simulink model "Proposed DTC"  (R2022a)
settings: Solver=ode1  StartTime=0.0  StopTime=Inf  FixedStep=Ts  RelTol=1e-3  EnableMultiTasking=on
PostLoadFcn:
  | , if any(exist('dsrtsu_mdlpostloadfcn', 'file') ~= 0), dsrtsu_mdlpostloadfcn('Execute', bdroot); end,
InitFcn:
  | , if any(exist('rtifpga_mdlclblib', 'file') ~= 0), rtifpga_mdlclblib('Init', bdroot); end,
undefined symbols (not defined in the file): P, Ts
libraries: rtilib1104 x15, rtitasklib x1
(part 1 of 2)
settings Model: DSRTSU_INTERNAL_RTI_VER=600  DSRTSU_INTERNAL_RTI_TYPE=rti1104  DSRTSU_INTERNAL_RTIFPGA=180  DSRTSU_INTERNAL_RTISTBM_VER=1.4.4  Creator=Admin  LastModifiedBy=acer
settings SolverCC: AlgebraicLoopSolver=TrustRegion
settings DataIOCC: LimitDataPoints=on  SaveFormat=Array  SignalLoggingSaveFormat=ModelDataLogs  ReturnWorkspaceOutputs=off
settings OptimizationCC: BlockReduction=off  ConditionallyExecuteInputs=off  OptimizeBlockIOStorage=off  BufferReuse=off  GlobalBufferReuse=off  ExpressionFolding=off  ExpressionDepthLimit=2147483647  LocalBlockOutputs=off  LifeSpan=inf
settings DebuggingCC: UnderspecifiedInitializationDetection=Classic  MergeDetectMultiDrivingBlocksExec=none  SolverPrmCheckMsg=warning  MultiTaskDSMMsg=warning  MultiTaskCondExecSysMsg=none  FcnCallInpInsideContextMsg=warning  UnconnectedInputMsg=warning  UnconnectedOutputMsg=warning  UnconnectedLineMsg=warning  StateNameClashWarn=warning  SFUnexpectedBacktrackingDiag=warning  SFNoUnconditionalDefaultTransitionDiag=warning  SFExecutionAtInitializationDiag=none  SFMachineParentedDataDiag=warning  ArithmeticOperatorsInVariantConditions=warning
settings HardwareCC: ProdBitPerPointer=32  ProdBitPerSizeT=32  ProdBitPerPtrDiffT=32  ProdLargestAtomicInteger=Integer  ProdEndianess=BigEndian  ProdWordSize=32  ProdHWDeviceType=Custom Processor->Custom  TargetIntDivRoundTo=Zero  TargetEndianess=BigEndian  TargetHWDeviceType=Custom Processor->Custom
settings ModelReferenceCC: PropagateSignalLabelsOutOfModel=off
settings SFSimCC: SimUseLocalCustomCode=off  MATLABDynamicMemAlloc=off  CustomCodeUndefinedFunction=UseInterfaceOnly
settings RTWCC: Description=dSPACE DS1104 Hardware Platform  SystemTargetFile=rti1104.tlc  MakeCommand=make_rti  TemplateMakefile=rti1104.tmf  RTWUseLocalCustomCode=off
settings CodeAppCC: StateflowObjectComments=on
settings STFCustomTargetCC: ParMdlRefBuildCompliant=on  GRTInterface=off  SystemTargetFile=rti1104.tlc
settings GRTTargetCC: TargetLangStandard=C89/C90 (ANSI)  CompOptLevelCompliant=off  ConcurrentExecutionCompliant=off  CombineOutputUpdateFcns=off  MatFileLogging=off  CPPClassGenCompliant=off  UseToolchainInfoCompliant=off  ExtModeMexFile=noextcomm
settings ConfigComp: CovMetricSettings=dw  CovSaveCumulativeToWorkspaceVar=on  CovSaveSingleToWorkspaceVar=on  CovExternalEMLEnable=off

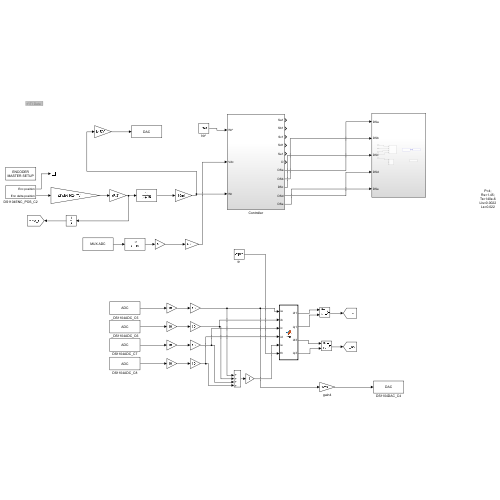
[thumbnail: Simulink's stored preview of the top-level diagram]
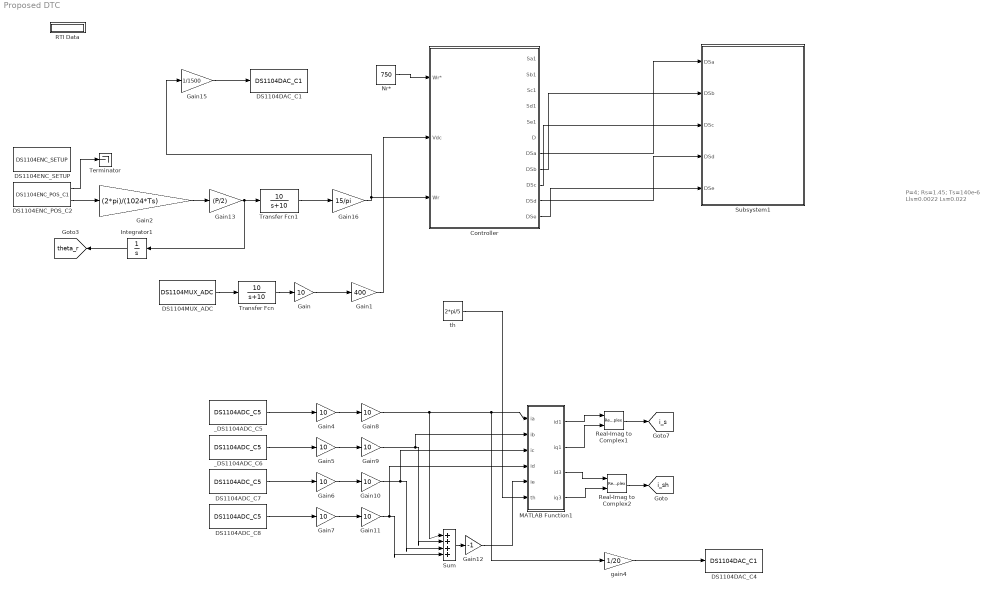
== system Proposed DTC ==
  note: P=4;
      | Rs=1.45;
      | Ts=140e-6
      | Lls=0.0022
      | Ls=0.022
  Controller : Subsystem
  DS1104ADC_C7 : rtilib1104/DS1104 MASTER PPC/DS1104ADC_C5  ChannelNo=7  TriggerMode=0  Reserved1=[]  Reserved2=[]  Reserved3=[]  Reserved4=[]  DialogFcn=gui1104adc  UnitName={ 'DS1104ADC_C' }  UnitValues={ 7 }  DSProperties=struct('RTI',struct('Version',uint32(1),'BlockType',struct('isSLSource',uint8(1),'isSLSink',uint8(0),'isHWSource',uint8(1),'isHWSink',uint8(0),'isSetup',uint8(0),'isInline',uint8(1),'isNonInline',uint8(0),'isInterrupt',uint8(0),'isChannelwise',uint8(1)),'IOBoardType','DS1104MASTER','UnitType','ADC','Identifier','ADC','DialogType','ML','BlockSet','NONE','SlaveProcessor','NONE'))
      settings: SourceProductName=dSPACE RTI1104
  DS1104ADC_C8 : rtilib1104/DS1104 MASTER PPC/DS1104ADC_C5  ChannelNo=8  TriggerMode=0  Reserved1=[]  Reserved2=[]  Reserved3=[]  Reserved4=[]  DialogFcn=gui1104adc  UnitName={ 'DS1104ADC_C' }  UnitValues={ 8 }  DSProperties=struct('RTI',struct('Version',uint32(1),'BlockType',struct('isSLSource',uint8(1),'isSLSink',uint8(0),'isHWSource',uint8(1),'isHWSink',uint8(0),'isSetup',uint8(0),'isInline',uint8(1),'isNonInline',uint8(0),'isInterrupt',uint8(0),'isChannelwise',uint8(1)),'IOBoardType','DS1104MASTER','UnitType','ADC','Identifier','ADC','DialogType','ML','BlockSet','NONE','SlaveProcessor','NONE'))
      settings: SourceProductName=dSPACE RTI1104
  DS1104DAC_C1 : rtilib1104/DS1104 MASTER PPC/DS1104DAC_C1  ChannelNo=1  InitValue=0  TermMode=0  TermValue=0  Reserved1=[]  Reserved2=[]  Reserved3=[]  Reserved4=[]  DialogFcn=gui1104dac  UnitName={ 'DS1104DAC_C'}  UnitValues={ 1 }  DSProperties=struct('RTI',struct('Version',uint32(1),'BlockType',struct('isSLSource',uint8(0),'isSLSink',uint8(1),'isHWSource',uint8(0),'isHWSink',uint8(1),'isSetup',uint8(0),'isInline',uint8(1),'isNonInline',uint8(0),'isInterrupt',uint8(0),'isChannelwise',uint8(1)),'IOBoardType','DS1104MASTER','UnitType','DAC','Identifier','DAC','DialogType','ML','BlockSet','NONE','SlaveProcessor','NONE'))
      settings: SourceProductName=dSPACE RTI1104
  DS1104DAC_C4 : rtilib1104/DS1104 MASTER PPC/DS1104DAC_C1  ChannelNo=4  InitValue=0  TermMode=0  TermValue=0  Reserved1=[]  Reserved2=[]  Reserved3=[]  Reserved4=[]  DialogFcn=gui1104dac  UnitName={ 'DS1104DAC_C'}  UnitValues={4}  DSProperties=struct('RTI',struct('Version',uint32(1),'BlockType',struct('isSLSource',uint8(0),'isSLSink',uint8(1),'isHWSource',uint8(0),'isHWSink',uint8(1),'isSetup',uint8(0),'isInline',uint8(1),'isNonInline',uint8(0),'isInterrupt',uint8(0),'isChannelwise',uint8(1)),'IOBoardType','DS1104MASTER','UnitType','DAC','Identifier','DAC','DialogType','ML','BlockSet','NONE','SlaveProcessor','NONE'))
      settings: SourceProductName=dSPACE RTI1104
  DS1104ENC_POS_C2 : rtilib1104/DS1104 MASTER PPC/DS1104ENC_POS_C1  ChannelNo=2  PosValue=0  Reserved1=[]  Reserved2=[]  Reserved3=[]  Reserved4=[]  DialogFcn=gui1104enc_pos  UnitName={'DS1104ENC_POS_C'}  UnitValues={ 2 }  DSProperties=struct('RTI',struct('Version',uint32(1),'BlockType',struct('isSLSource',uint8(1),'isSLSink',uint8(0),'isHWSource',uint8(1),'isHWSink',uint8(0),'isSetup',uint8(0),'isInline',uint8(1),'isNonInline',uint8(0),'isInterrupt',uint8(0),'isChannelwise',uint8(1)),'IOBoardType','DS1104MASTER','UnitType','ENC','Identifier','ENCPOSCH','DialogType','ML','BlockSet','NONE','SlaveProcessor','NONE'))
      settings: SourceProductName=dSPACE RTI1104
  DS1104ENC_SETUP : rtilib1104/DS1104 MASTER PPC/DS1104ENC_SETUP  Reserved1=[]  Reserved2=[]  Reserved3=[]  Reserved4=[]  DialogFcn=gui1104enc_setup  UnitName={'DS1104ENC_SETUP'}  UnitValues={ [] }  DSProperties=struct('RTI',struct('Version',uint32(1),'BlockType',struct('isSLSource',uint8(0),'isSLSink',uint8(0),'isHWSource',uint8(0),'isHWSink',uint8(0),'isSetup',uint8(0),'isInline',uint8(1),'isNonInline',uint8(0),'isInterrupt',uint8(0),'isChannelwise',uint8(0)),'IOBoardType','DS1104MASTER','UnitType','ENC','Identifier','ENCSETUP','DialogType','ML','BlockSet','NONE','SlaveProcessor','NONE'))
      settings: SourceProductName=dSPACE RTI1104  SignalType=[0 0]
  DS1104MUX_ADC : rtilib1104/DS1104 MASTER PPC/DS1104MUX_ADC  ChannelNos=1  TriggerMode=0  Reserved1=[]  Reserved2=[]  Reserved3=[]  Reserved4=[]  DialogFcn=gui1104mux_adc  UnitName={ 'DS1104MUX_ADC' }  UnitValues={ [] }  DSProperties=struct('RTI',struct('Version',uint32(1),'BlockType',struct('isSLSource',uint8(1),'isSLSink',uint8(0),'isHWSource',uint8(1),'isHWSink',uint8(0),'isSetup',uint8(0),'isInline',uint8(1),'isNonInline',uint8(0),'isInterrupt',uint8(0),'isChannelwise',uint8(0)),'IOBoardType','DS1104MASTER','UnitType','ADC','Identifier','ADCMUX','DialogType','ML','BlockSet','NONE','SlaveProcessor','NONE'))
      settings: SourceProductName=dSPACE RTI1104
  Gain{,4..11} (9 alike) : Gain  Gain=10
  Gain1 : Gain  Gain=400
  Gain12 : Gain  Gain=-1
  Gain13 : Gain  Gain=(P/2)
  Gain15 : Gain  Gain=1/1500
  Gain16 : Gain  Gain=15/pi
  Gain2 : Gain  Gain=(2*pi)/(1024*Ts)
  Integrator1 : Integrator  UpperSaturationLimit=30  LowerSaturationLimit=-30
  MATLAB Function1 : MATLAB Function  TreatAsAtomicUnit=on
  Nr* : Constant  Value=750
  RTI Data : Subsystem  Tag=struct('RTIDataServer',struct('RTIDataServerVs','2','RTIModelDescription','struct(''main'',''Proposed_DTC_PWMnD_2ndway'',''sub'','''',''isMp'',0)'))  LoadFcn="if exist('rtidc'), try,  rtidc('DataHostBlockClbLoad', gcbh); catch, disp(['Warning: ''LoadFcn'' for RTI Data block failed: ' lasterr]); end, end,"  mask(RTI_DATA_HOST){}
      mask help:
      | RTI Data Block.
      | This block is used by RTI to store internal model-dependent data.
      | Please keep this block on the root level of the model. Deleting this block will result in data loss.
      |
      | NEVER DELETE OR COPY THIS BLOCK!
      settings: CopyFcn="if exist('rtidc'), try,  rtidc('DataHostBlockClbCopy', gcbh); catch, disp(['Warning: ''CopyFcn'' for RTI Data block failed: ' lasterr]); end, end,"  DeleteFcn="if exist('rtidc'), try,  rtidc('DataHostBlockClbDelete', gcbh); catch, disp(['Warning: ''DeleteFcn'' for RTI Data block failed: ' lasterr]); end, end,"  ModelCloseFcn="if exist('rtidc'), try,  rtidc('DataHostBlockClbModelClose', gcbh); catch, disp(['Warning: ''ModelCloseFcn'' for RTI Data block failed: ' lasterr]); end, end,"  PreSaveFcn="if exist('rtidc'), try,  rtidc('DataHostBlockClbPreSave', gcbh); catch, disp(['Warning: ''PreSaveFcn'' for RTI Data block failed: ' lasterr]); end, end,"  PostSaveFcn="if exist('rtidc'), try,  rtidc('DataHostBlockClbPostSave', gcbh); catch, disp(['Warning: ''PostSaveFcn'' for RTI Data block failed: ' lasterr]); end, end,"  NameChangeFcn="if exist('rtidc'), try,  rtidc('DataHostBlockClbNameChange', gcbh); catch, disp(['Warning: ''NameChangeFcn'' for RTI Data block failed: ' lasterr]); end, end,"
      mask Help:
      | RTI Data Block.
      | This block is used by RTI to store internal model-dependent data.
      | Please keep this block on the root level of the model. Deleting this block will result in data loss.
      | 
      | NEVER DELETE OR COPY THIS BLOCK!
      mask Display:
      | text(0.5, 0.5, 'RTI Data', 'HorizontalAlignment', 'center');
      | plot([1 0]);
  Real-Imag to Complex1 : RealImagToComplex
  Real-Imag to Complex2 : RealImagToComplex
  Subsystem1 : Subsystem
  Sum : Sum  Inputs=|++++
  Terminator : Terminator
  Transfer Fcn : TransferFcn  Numerator=[10]  Denominator=[1 10]
  Transfer Fcn1 : TransferFcn  Numerator=[10]  Denominator=[1 10]
  _DS1104ADC_C5 : rtilib1104/DS1104 MASTER PPC/DS1104ADC_C5  ChannelNo=5  TriggerMode=0  Reserved1=[]  Reserved2=[]  Reserved3=[]  Reserved4=[]  DialogFcn=gui1104adc  UnitName={ 'DS1104ADC_C' }  UnitValues={ 5 }  DSProperties=struct('RTI',struct('Version',uint32(1),'BlockType',struct('isSLSource',uint8(1),'isSLSink',uint8(0),'isHWSource',uint8(1),'isHWSink',uint8(0),'isSetup',uint8(0),'isInline',uint8(1),'isNonInline',uint8(0),'isInterrupt',uint8(0),'isChannelwise',uint8(1)),'IOBoardType','DS1104MASTER','UnitType','ADC','Identifier','ADC','DialogType','ML','BlockSet','NONE','SlaveProcessor','NONE'))
      settings: SourceProductName=dSPACE RTI1104
  _DS1104ADC_C6 : rtilib1104/DS1104 MASTER PPC/DS1104ADC_C5  ChannelNo=6  TriggerMode=0  Reserved1=[]  Reserved2=[]  Reserved3=[]  Reserved4=[]  DialogFcn=gui1104adc  UnitName={ 'DS1104ADC_C' }  UnitValues={ 6 }  DSProperties=struct('RTI',struct('Version',uint32(1),'BlockType',struct('isSLSource',uint8(1),'isSLSink',uint8(0),'isHWSource',uint8(1),'isHWSink',uint8(0),'isSetup',uint8(0),'isInline',uint8(1),'isNonInline',uint8(0),'isInterrupt',uint8(0),'isChannelwise',uint8(1)),'IOBoardType','DS1104MASTER','UnitType','ADC','Identifier','ADC','DialogType','ML','BlockSet','NONE','SlaveProcessor','NONE'))
      settings: SourceProductName=dSPACE RTI1104
  gain4 : Gain  Gain=1/20  SaturateOnIntegerOverflow=on  OutDataTypeStr=Inherit: Same as input  ParamDataTypeStr=Inherit: Same as input
  th : Constant  Value=2*pi/5
  tag scope: i_s=global, i_sh=global, theta_r=global
  wires:
  th/1 -> MATLAB Function1/6(th)
  Gain12/1 -> MATLAB Function1/5(ie)
  Real-Imag to Complex2/1 -> [i_sh]
  _DS1104ADC_C5/1 -> Gain4/1
  Gain7/1 -> Gain11/1
  DS1104ADC_C8/1 -> Gain7/1
  Gain5/1 -> Gain9/1
  Gain9/1 -> MATLAB Function1/2(ib), Sum/2
  _DS1104ADC_C6/1 -> Gain5/1
  Gain1/1 -> Controller/2(Vdc)
  Nr*/1 -> Controller/1(Wr*)
  MATLAB Function1/4(iq3) -> Real-Imag to Complex2/2
  Gain10/1 -> MATLAB Function1/3(ic), Sum/3
  Transfer Fcn1/1 -> Gain16/1
  MATLAB Function1/2(iq1) -> Real-Imag to Complex1/2
  Integrator1/1 -> [theta_r]
  Transfer Fcn/1 -> Gain/1
  DS1104MUX_ADC/1 -> Transfer Fcn/1
  Gain/1 -> Gain1/1
  Gain13/1 -> Transfer Fcn1/1, Integrator1/1
  Sum/1 -> Gain12/1
  Gain4/1 -> Gain8/1
  Gain2/1 -> Gain13/1
  Gain6/1 -> Gain10/1
  DS1104ENC_POS_C2/2 -> Gain2/1
  Gain11/1 -> MATLAB Function1/4(id), Sum/4
  MATLAB Function1/3(id3) -> Real-Imag to Complex2/1
  MATLAB Function1/1(id1) -> Real-Imag to Complex1/1
  DS1104ADC_C7/1 -> Gain6/1
  DS1104ENC_POS_C2/1 -> Terminator/1
  Real-Imag to Complex1/1 -> [i_s]
  Gain16/1 -> Gain15/1, Controller/3(Wr)
  Gain15/1 -> DS1104DAC_C1/1
  gain4/1 -> DS1104DAC_C4/1
  Gain8/1 -> gain4/1, MATLAB Function1/1(ia), Sum/1
  Controller/7(DSa) -> Subsystem1/1(DSa)
  Controller/8(DSb) -> Subsystem1/2(DSb)
  Controller/9(DSc) -> Subsystem1/3(DSc)
  Controller/10(DSd) -> Subsystem1/4(DSd)
  Controller/11(DSe) -> Subsystem1/5(DSe)

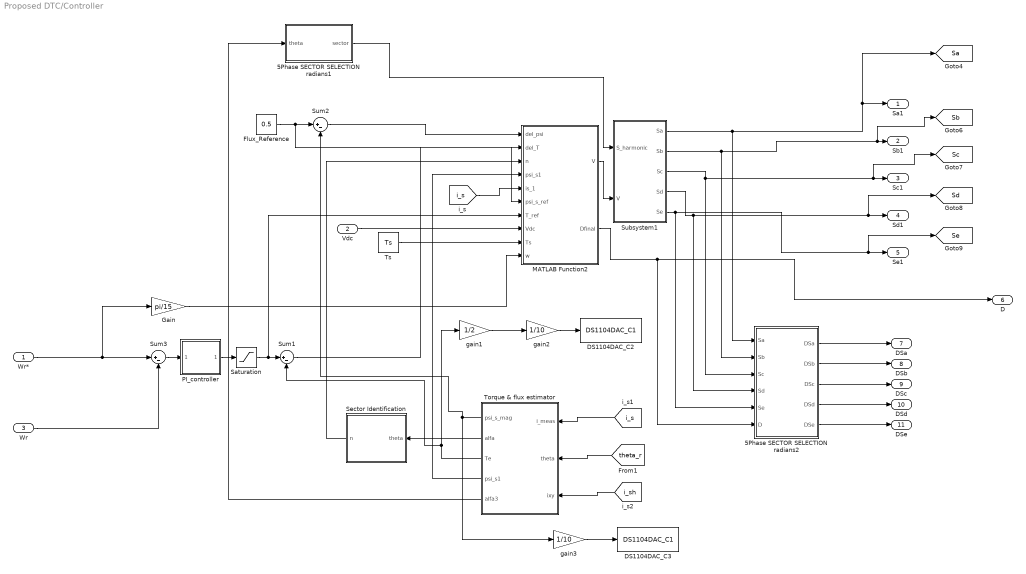
== system Proposed DTC/Controller ==
  Wr* : Inport
  Vdc : Inport  Port=2
  Wr : Inport  Port=3
  5Phase SECTOR SELECTION radians1 : MATLAB Function  TreatAsAtomicUnit=on
  5Phase SECTOR SELECTION radians2 : MATLAB Function  TreatAsAtomicUnit=on
  DS1104DAC_C2 : rtilib1104/DS1104 MASTER PPC/DS1104DAC_C1  ChannelNo=2  InitValue=0  TermMode=0  TermValue=0  Reserved1=[]  Reserved2=[]  Reserved3=[]  Reserved4=[]  DialogFcn=gui1104dac  UnitName={ 'DS1104DAC_C'}  UnitValues={ 2 }  DSProperties=struct('RTI',struct('Version',uint32(1),'BlockType',struct('isSLSource',uint8(0),'isSLSink',uint8(1),'isHWSource',uint8(0),'isHWSink',uint8(1),'isSetup',uint8(0),'isInline',uint8(1),'isNonInline',uint8(0),'isInterrupt',uint8(0),'isChannelwise',uint8(1)),'IOBoardType','DS1104MASTER','UnitType','DAC','Identifier','DAC','DialogType','ML','BlockSet','NONE','SlaveProcessor','NONE'))
      settings: SourceProductName=dSPACE RTI1104
  DS1104DAC_C3 : rtilib1104/DS1104 MASTER PPC/DS1104DAC_C1  ChannelNo=3  InitValue=0  TermMode=0  TermValue=0  Reserved1=[]  Reserved2=[]  Reserved3=[]  Reserved4=[]  DialogFcn=gui1104dac  UnitName={ 'DS1104DAC_C'}  UnitValues={ 3 }  DSProperties=struct('RTI',struct('Version',uint32(1),'BlockType',struct('isSLSource',uint8(0),'isSLSink',uint8(1),'isHWSource',uint8(0),'isHWSink',uint8(1),'isSetup',uint8(0),'isInline',uint8(1),'isNonInline',uint8(0),'isInterrupt',uint8(0),'isChannelwise',uint8(1)),'IOBoardType','DS1104MASTER','UnitType','DAC','Identifier','DAC','DialogType','ML','BlockSet','NONE','SlaveProcessor','NONE'))
      settings: SourceProductName=dSPACE RTI1104
  Flux_Reference : Constant  Value=0.5
  Gain : Gain  Gain=pi/15
  MATLAB Function2 : MATLAB Function  TreatAsAtomicUnit=on  SystemSampleTime=Ts
  PI_controller : Subsystem
  Saturation : Saturate  UpperLimit=14  LowerLimit=-14
  Sector Identification : MATLAB Function  TreatAsAtomicUnit=on  SystemSampleTime=Ts
  Subsystem1 : Subsystem
  Sum1 : Sum  Inputs=|+-
  Sum2 : Sum  Inputs=|+-
  Sum3 : Sum  Inputs=|+-
  Torque & flux estimator : MATLAB Function  TreatAsAtomicUnit=on  SystemSampleTime=Ts
  Ts : Constant  Value=Ts
  gain1 : Gain  Gain=1/2  SaturateOnIntegerOverflow=on  OutDataTypeStr=Inherit: Same as input  ParamDataTypeStr=Inherit: Same as input
  gain2 : Gain  Gain=1/10  SaturateOnIntegerOverflow=on  OutDataTypeStr=Inherit: Same as input  ParamDataTypeStr=Inherit: Same as input
  gain3 : Gain  Gain=1/10  SaturateOnIntegerOverflow=on  OutDataTypeStr=Inherit: Same as input  ParamDataTypeStr=Inherit: Same as input
  Sa1 : Outport
  Sb1 : Outport  Port=2
  Sc1 : Outport  Port=3
  Sd1 : Outport  Port=4
  Se1 : Outport  Port=5
  D : Outport  Port=6
  DSa : Outport  Port=7
  DSb : Outport  Port=8
  DSc : Outport  Port=9
  DSd : Outport  Port=10
  DSe : Outport  Port=11
  tag scope: Sa=global, Sb=global, Sc=global, Sd=global, Se=global
  wires:
  [theta_r] -> Torque & flux estimator/2(theta)
  Torque & flux estimator/2(alfa) -> Sector Identification/1(theta)
  Wr*/1 -> Gain/1, Sum3/1
  PI_controller/1(PI_out) -> Saturation/1
  Wr/1 -> Sum3/2
  [i_s] -> Torque & flux estimator/1(i_meas)
  Sum3/1 -> PI_controller/1(error)
  Flux_Reference/1 -> MATLAB Function2/6(psi_s_ref), Sum2/1
  Saturation/1 -> MATLAB Function2/7(T_ref), Sum1/1
  Ts/1 -> MATLAB Function2/9(Ts)
  Torque & flux estimator/4(psi_s1) -> MATLAB Function2/4(psi_s1)
  [i_s] -> MATLAB Function2/5(is_1)
  Sector Identification/1(n) -> MATLAB Function2/3(n)
  Sum1/1 -> MATLAB Function2/2(del_T)
  Sum2/1 -> MATLAB Function2/1(del_psi)
  MATLAB Function2/1(V) -> Subsystem1/2(V)
  5Phase SECTOR SELECTION radians1/1(sector) -> Subsystem1/1(S_harmonic)
  Vdc/1 -> MATLAB Function2/8(Vdc)
  Torque & flux estimator/5(alfa3) -> 5Phase SECTOR SELECTION radians1/1(theta)
  Subsystem1/1(Sa) -> 5Phase SECTOR SELECTION radians2/1(Sa), [Sa], Sa1/1
  Subsystem1/3(Sc) -> 5Phase SECTOR SELECTION radians2/3(Sc), [Sc], Sc1/1
  Subsystem1/4(Sd) -> 5Phase SECTOR SELECTION radians2/4(Sd), [Sd], Sd1/1
  Subsystem1/5(Se) -> 5Phase SECTOR SELECTION radians2/5(Se), [Se], Se1/1
  Subsystem1/2(Sb) -> 5Phase SECTOR SELECTION radians2/2(Sb), [Sb], Sb1/1
  MATLAB Function2/2(Dfinal) -> 5Phase SECTOR SELECTION radians2/6(D), D/1
  Gain/1 -> MATLAB Function2/10(w)
  5Phase SECTOR SELECTION radians2/1(DSa) -> DSa/1
  5Phase SECTOR SELECTION radians2/2(DSb) -> DSb/1
  5Phase SECTOR SELECTION radians2/3(DSc) -> DSc/1
  5Phase SECTOR SELECTION radians2/4(DSd) -> DSd/1
  5Phase SECTOR SELECTION radians2/5(DSe) -> DSe/1
  gain2/1 -> DS1104DAC_C2/1
  Torque & flux estimator/3(Te) -> gain1/1, Sum1/2
  gain1/1 -> gain2/1
  gain3/1 -> DS1104DAC_C3/1
  Torque & flux estimator/1(psi_s_mag) -> Sum2/2, gain3/1
  [i_sh] -> Torque & flux estimator/3(ixy)

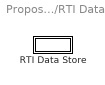
== system Proposed DTC/RTI Data ==
  RTI Data Store : Subsystem  Tag="struct('private',struct('version',struct('dsVer',uint32(2),'dsVerCreation',uint32(2),'RTI',struct('ver','7.18','type','RTI1104')),'access',struct('type','Model','isPerm',1,'created',['03-Apr-2024 11:27:50'],'modified',['16-Aug-2024 21:38:16'],'location','')),'public',struct('main',struct('data',[]),'sub',struct('name',{{'Proposed_DTC_PWMnD_2ndway'}},'data',{{struct('TH',struct('thTaskInfo',struct('taskType',{'TIMER','HWINT','TMRINT','SWINT','GLINT'},'tasksNumOf',{1,0,0,0,0},'srcIds',{{'PWMINT'},{},{},{},{}},'taskNames',{{['Timer Task 1']},{},{},{},{}})),'th_tc',struct('dataType','TASK','taskGroupId','','taskGroupList',{{}},'taskSchedulingPolicy','FCFS','taskType','TIMER','blkh','Proposed_DTC_PWMnD_2ndway/Subsystem1/DS1104SLAVE_PWMINT1','srcId','PWMINT','srcSgnName',['SLAVE-PWM-Interrupt with variable alignment'],'srcCpuName','','taskName',['Timer Task 1  [0.00014] s'],'taskNameDisplayExt','','smplTime',0.00014,'smplTimeOffs',0,'hasFixedPriority',0,'priority',1,'hasFixedOvc',0,'ovcType',1,'ovcMax',1),'tc_th',struct('dataType','TASK','taskGroupId','','taskGroupList',{{}},'taskSchedulingPolicy','FCFS','taskType','TIMER','blkh','Proposed_DTC_PWMnD_2ndway/Subsystem1/DS1104SLAVE_PWMINT1','srcId','PWMINT','srcSgnName',['SLAVE-PWM-Interrupt with variable alignment'],'srcCpuName','','taskName',['Timer Task 1  [0.00014] s'],'taskNameDisplayExt','','smplTime',0.00014,'smplTimeOffs',0,'hasFixedPriority',0,'priority',1,'hasFixedOvc',0,'ovcType',1,'ovcMax',1))}})))"  mask(RTI_DATA_STORE){}
      mask help:
      | RTI Data Store Block. This block is used by RTI to store internal model dependent data. Deleting this block will result in data loss.
      |
      | NEVER DELETE, COPY, OR MODIFY THIS BLOCK!
      mask Help:
      | RTI Data Store Block. This block is used by RTI to store internal model dependent data. Deleting this block will result in data loss.
      | 
      | NEVER DELETE, COPY, OR MODIFY THIS BLOCK!
      mask Display: text(0.5, 0.5, ' ', 'HorizontalAlignment', 'center');

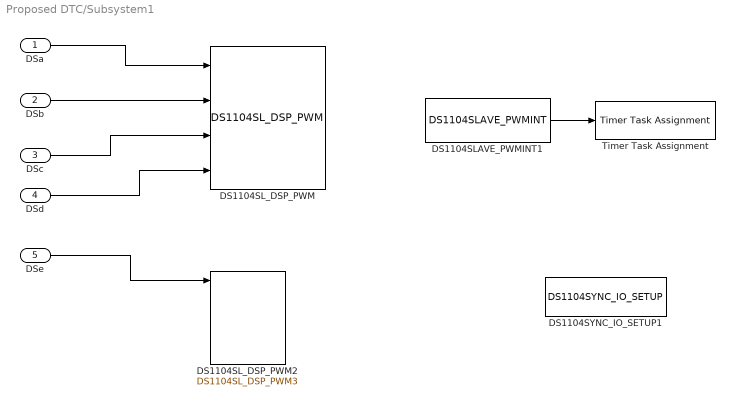
== system Proposed DTC/Subsystem1 ==
  DSa : Inport
  DSb : Inport  Port=2
  DSc : Inport  Port=3
  DSd : Inport  Port=4
  DSe : Inport  Port=5
  DS1104SLAVE_PWMINT1 : rtilib1104/DS1104 SLAVE DSP/DS1104SLAVE_PWMINT  Parameters=[]  TDef=[]  BoardIntNo=[]  InterruptName=[]  Delay=[]  DialogFcn=[]  Reserved1=[]  Reserved2=[]  Reserved3=[]  Reserved4=[]  Revision=[]  UnitName=[]  UnitValues=[]  DSProperties=struct('RTI',struct('Version',uint32(530),'IOBoardType','DS1104SLAVE','SlaveProcessor','F240','UnitType','HWINT','Identifier','PWMINT','BlockType',struct('isSLSource',uint8(1),'isSLSink',uint8(0),'isHWSource',uint8(1),'isHWSink',uint8(0),'isSetup',uint8(0),'isInline',uint8(1),'isNonInline',uint8(0),'isInterrupt',uint8(1),'isChannelwise',uint8(0)),'DialogType','ML','BlockSet','NONE','RelationId',struct('TH',struct('BlockId','HWINT'))))  RTIBlockInterface=struct('BlockName',struct('Token',{{'DS1104SLAVE_PWMINT'}}),'BlockDisplay',{{['DS1104SLAVE Board \nPWM-Interrupt'],'center'}},'DialogFcn','rti110xhwintgui','OutputPortsActive',1,'OutputPortsWidth',int32(1),'FunctionCall',uint32(0),'OutputPortsName',{{[' ']}},'IconTransparency','on','InitLevel',3,'Options',{{'SS_OPTION_FORCE_NONINLINED_FCNCALL','SS_OPTION_ASYNCHRONOUS_INTERRUPT'}},'OutputPortsDataType',{{'SS_FCN_CALL'}})  RTIBlockParameters=struct('ThIntNo',{{10,'OFF',[]}},'IntDelay',{{0.01,'ON',[1e-6 1]}},'ThSrcSgnName',{{['SLAVE-PWM-Interrupt with variable alignment'],'OFF',[]}},'TLCFileName',{{'rti1104slave_pwm_interrupt','OFF',[]}},'ThBlk',{{['struct(''blkh'',''Proposed_DTC_PWMnD_2ndway/Subsystem1/DS1104SLAVE_PWMINT1'',''srcId'',''PWMINT'',''srcSgnId'',''PWMINT'',''intervalTmrBlockId'',[],''srcSgnName'',[''SLAVE-PWM-Interrupt with variable alignment''],''srcCpuId'','''',''isSrcCpu'',1,''isTargetCpu'',1,''srcOnMasterCpu'',1,''boardType'','''',''boardTypeNo'','''',''boardNo'',1,''intNo'',0,''subIntNo'',-1,''period'',0,''entryPoint'',''rti_PWMINT'',''blockName'',''DS1104SLAVE_PWMINT1'',''taskNameDisplayExt'','''',''taskType'',''HWINT'',''groupId'',''PWMINT'',''hookFcn'',''NULL'',''isTimerTaskSrc'',1,''service'','''',''mpBlkId'','''',''taskPriorityPreConfig'',''none'',''taskPriority'',-1,''taskSortWeighting'',[],''taskSchedulingPolicy'',''FCFS'',''taskOvrPreConfig'',''none'',''taskOvrStrategy'',1,''taskOvrQueueSize'',1,''taskVisibility'',''on'',''taskGroupId'','''',''taskGroupDisplayOrder'',[],''serviceDynamicGen'',0,''disableCodeGen'',0,''boardBase'',''0'',''noBoardBase'','''')'],'OFF',[]}},'PHSBoardBaseId',{{'DSXXXX','OFF',[]}})  RTISFcnParameters=struct('IntDelay','double','ThBlk','struct','ThIntNo','int32','TLCFileName','char','PHSBoardBaseId','char')  RTIBlockParaDefault=struct('ThIntNo',10,'IntDelay',2^-1,'ThSrcSgnName',['SLAVE-PWM-Interrupt with none delay'],'TLCFileName','rti1104slave_pwm_interrupt','ThBlk',['struct(''srcSgnId'', '''')'],'PHSBoardBaseId','DSXXXX')
      settings: SourceProductName=dSPACE RTI1104
  DS1104SL_DSP_PWM : rtilib1104/DS1104 SLAVE DSP/DS1104SL_DSP_PWM  Parameters=[]  TDef=[]  BoardType=[]  PwmMode=[]  Frequency=[]  InitValue=[]  TermMode=[]  TermValue=[]  Polarity=[]  DialogFcn=[]  Reserved1=[]  Reserved2=[]  Reserved3=[]  Reserved4=[]  Revision=[]  UnitName=[]  UnitValues=[]  DSProperties=struct('RTI',struct('Version',uint32(2),'BlockType',struct('isSLSource',uint8(0),'isSLSink',uint8(1),'isHWSource',uint8(0),'isHWSink',uint8(1),'isSetup',uint8(0),'isInline',uint8(1),'isNonInline',uint8(0),'isInterrupt',uint8(0),'isChannelwise',uint8(0)),'IOBoardType','DS1104SLAVE','UnitType','PWM','Identifier','PWM','DialogType','ML','BlockSet','NONE','SlaveProcessor','F240'))  RTIBlockInterface=struct('InputPortsActive',[1 1 1 1],'InputPortsWidth',int32([1 1 1 1]),'InputPortsName',{{['PWM Channel 1'],['PWM Channel 2'],['PWM Channel 3'],['PWM Channel 4']}},'IWork',{{{'',uint32(4)}}},'DialogFcn','rti1104slavepwmgui','InitLevel',1,'BlockDisplay',{{'','auto'}},'IconTransparency','on','MultiSFcn',4,'BlockName',struct('Token',{{'DS1104SL_DSP_PWM'}}))  RTIBlockParameters=struct('PWMSymmetryMode',{{1,'OFF',[]}},'PWMFrequency',{{'1/Ts','OFF',[]}},'PWMPolarityMode',{{[1 1 1 1 1],'OFF',[]}},'ChannelNo',{{[1 2 3 4],'OFF',[]}},'SuspendModeInit',{{[1 1 1 1 1],'OFF',[]}},'TTLModeInit',{{[2 2 2 2 2],'OFF',[]}},'DutyCycleInitValueCh1',{{'0.5','OFF',[]}},'DutyCycleInitValueCh2',{{'0.5','OFF',[]}},'DutyCycleInitValueCh3',{{'0.5','OFF',[]}},'DutyCycleInitValueCh4',{{'0.5','OFF',[]}},'DutyCycleInitValueCh5',{{'0.5','OFF',[]}},'EnablePWMStop',{{[0 0 0 0 0],'OFF',[]}},'SuspendModeTerm',{{[0 1 1 1 1],'OFF',[]}},'TTLModeTerm',{{[2 2 2 2 2],'OFF',[]}},'DutyCycleTermValueCh1',{{'0.5','OFF',[]}},'DutyCycleTermValueCh2',{{'0.5','OFF',[]}},'DutyCycleTermValueCh3',{{'0.5','OFF',[]}},'DutyCycleTermValueCh4',{{'0.5','OFF',[]}},'DutyCycleTermValueCh5',{{'0.5','OFF',[]}},'TLCFileName',{{'rti1104pwm','OFF',[]}})  RTISFcnParameters=struct('PWMSymmetryMode','double','PWMFrequency','double','PWMPolarityMode','double','ChannelNo','double','SuspendModeInit','double','TTLModeInit','double','DutyCycleInitValueCh1','double','DutyCycleInitValueCh2','double','DutyCycleInitValueCh3','double','DutyCycleInitValueCh4','double','EnablePWMStop','double','SuspendModeTerm','double','TTLModeTerm','double','DutyCycleTermValueCh1','double','DutyCycleTermValueCh2','double','DutyCycleTermValueCh3','double','DutyCycleTermValueCh4','double','TLCFileName','char')  RTIBlockParaDefault=struct('PWMSymmetryMode',1,'PWMFrequency',100,'PWMPolarityMode',[1 1 1 1 1],'ChannelNo',[1 2 3 4],'SuspendModeInit',[1 1 1 1 1],'TTLModeInit',[2 2 2 2 2],'DutyCycleInitValueCh1',2^-1,'DutyCycleInitValueCh2',2^-1,'DutyCycleInitValueCh3',2^-1,'DutyCycleInitValueCh4',2^-1,'DutyCycleInitValueCh5',2^-1,'EnablePWMStop',[1 1 1 1 0],'SuspendModeTerm',[1 1 1 1 1],'TTLModeTerm',[2 2 2 2 2],'DutyCycleTermValueCh1',2^-1,'DutyCycleTermValueCh2',2^-1,'DutyCycleTermValueCh3',2^-1,'DutyCycleTermValueCh4',2^-1,'DutyCycleTermValueCh5',2^-1,'TLCFileName','rti1104pwm')
      settings: SourceProductName=dSPACE RTI1104
  DS1104SL_DSP_PWM2 : rtilib1104/DS1104 SLAVE DSP/DS1104SL_DSP_PWM3  Parameters=[]  TDef=[]  BoardType=[]  PwmMode=[]  Frequency=[]  DeadBand=[]  InitValue=[]  TermMode=[]  TermValue=[]  IntDelay=[]  DialogFcn=[]  Reserved1=[]  Reserved2=[]  Reserved3=[]  Reserved4=[]  Revision=[]  UnitName=[]  UnitValues=[]  DSProperties=struct('RTI',struct('Version',uint32(2),'BlockType',struct('isSLSource',uint8(0),'isSLSink',uint8(1),'isHWSource',uint8(0),'isHWSink',uint8(1),'isSetup',uint8(0),'isInline',uint8(1),'isNonInline',uint8(0),'isInterrupt',uint8(0),'isChannelwise',uint8(0)),'IOBoardType','DS1104SLAVE','UnitType','PWM','Identifier','PWM3','DialogType','ML','BlockSet','NONE','SlaveProcessor','F240'))  RTIBlockInterface=struct('InputPortsActive',[1 1 1 1],'InputPortsWidth',int32([1 1 1 1]),'InputPortsName',{{['Duty cycle a'],['Duty cycle b'],['Duty cycle c'],['PWM Stop']}},'IWork',{{{'',uint32(1)}}},'DialogFcn','rti1104slavepwm3gui','InitLevel',1,'BlockDisplay',{{'','auto'}},'IconTransparency','on','BlockName',struct('Token',{{'DS1104SL_DSP_PWM3'}}))  RTIBlockParameters=struct('PWMFrequency',{{'1/Ts','OFF',[]}},'PWMDeadband',{{'0','OFF',[]}},'PWMPolarityMode',{{[1 1 1 1],'OFF',[]}},'PWMPolarityInvMode',{{[2 2 2 2],'OFF',[]}},'SuspendModeInit',{{[1 1 1],'OFF',[]}},'TTLModeInit',{{[2 2 2],'OFF',[]}},'TTLModeInitNOT',{{[1 1 1],'OFF',[]}},'DutyCycleInitValueCh1',{{'0.5','OFF',[]}},'DutyCycleInitValueCh2',{{'0.5','OFF',[]}},'DutyCycleInitValueCh3',{{'0.5','OFF',[]}},'EnablePWMStop',{{1,'OFF',[]}},'SuspendModeTerm',{{[1 1 1],'OFF',[]}},'TTLModeTerm',{{[2 2 2],'OFF',[]}},'TTLModeTermNOT',{{[1 1 1],'OFF',[]}},'DutyCycleTermValueCh1',{{'0.5','OFF',[]}},'DutyCycleTermValueCh2',{{'0.5','OFF',[]}},'DutyCycleTermValueCh3',{{'0.5','OFF',[]}},'TLCFileName',{{'rti1104pwm3','OFF',[]}})  RTISFcnParameters=struct('PWMFrequency','double','PWMDeadband','double','PWMPolarityMode','double','PWMPolarityInvMode','double','SuspendModeInit','double','TTLModeInit','double','TTLModeInitNOT','double','DutyCycleInitValueCh1','double','DutyCycleInitValueCh2','double','DutyCycleInitValueCh3','double','EnablePWMStop','double','SuspendModeTerm','double','TTLModeTerm','double','TTLModeTermNOT','double','DutyCycleTermValueCh1','double','DutyCycleTermValueCh2','double','DutyCycleTermValueCh3','double','TLCFileName','char')  RTIBlockParaDefault=struct('PWMFrequency',100,'PWMDeadband',50,'PWMPolarityMode',[1 1 1 1],'PWMPolarityInvMode',[2 2 2 2],'SuspendModeInit',[1 1 1],'TTLModeInit',[2 2 2],'TTLModeInitNOT',[1 1 1],'DutyCycleInitValueCh1',2^-1,'DutyCycleInitValueCh2',2^-1,'DutyCycleInitValueCh3',2^-1,'EnablePWMStop',1,'SuspendModeTerm',[1 1 1],'TTLModeTerm',[2 2 2],'TTLModeTermNOT',[1 1 1],'DutyCycleTermValueCh1',2^-1,'DutyCycleTermValueCh2',2^-1,'DutyCycleTermValueCh3',2^-1,'TLCFileName','rti1104pwm3')
      settings: SourceProductName=dSPACE RTI1104
  DS1104SYNC_IO_SETUP1 : rtilib1104/DS1104 MASTER PPC/DS1104SYNC_IO_SETUP  DSProperties=struct('RTI',struct('Version',uint32(1),'BlockType',struct('isSLSource',uint8(0),'isSLSink',uint8(0),'isHWSource',uint8(0),'isHWSink',uint8(0),'isSetup',uint8(1),'isInline',uint8(1),'isNonInline',uint8(0),'isInterrupt',uint8(0),'isChannelwise',uint8(0)),'IOBoardType','DS1104MASTER','UnitType','SETUP','Identifier','SYNCSETUP','DialogType','ML','BlockSet','NONE','SlaveProcessor','NONE'))  RTIBlockInterface=struct('OutputPortsActive',0,'OutputPortsWidth',int32(0),'DialogFcn','gui1104mastersyncsetup','InitLevel',1,'BlockDisplay',{{['Master Sync IO Setup'],'center'}},'IconTransparency','off','BlockName',struct('Token',{{'DS1104SYNC_IO_SETUP'}}))  RTIBlockParameters=struct('TriggerSource',{{1,'OFF',[]}},'SyncIn',{{2,'OFF',[]}},'SyncOut',{{2,'OFF',[]}},'SyncADC',{{[0 0 0 0 0],'OFF',[]}},'SyncDAC',{{0,'OFF',[]}},'SyncInc',{{[0 0],'OFF',[]}},'TLCFileName',{{'rti1104mastersyncsetup','OFF',[]}})  RTISFcnParameters=struct('TriggerSource','int32','SyncIn','int32','SyncOut','int32','SyncADC','int32','SyncDAC','int32','SyncInc','int32','TLCFileName','char')  RTIBlockParaDefault=struct('TriggerSource',1,'SyncIn',1,'SyncOut',1,'SyncADC',[0 0 0 0 0],'SyncDAC',0,'SyncInc',[0 0],'TLCFileName','rti1104mastersyncsetup')
      settings: SourceProductName=dSPACE RTI1104
  Timer Task Assignment : rtitasklib/Timer Task Assignment  Reserved2=[]  Reserved3=[]  Reserved4=[]  DSProperties=struct('RTI',struct('Version',uint32(2),'BlockType',struct('isSLSource',uint8(0),'isSLSink',uint8(1),'isHWSource',uint8(0),'isHWSink',uint8(0),'isSetup',uint8(0),'isInline',uint8(1),'isNonInline',uint8(0),'isInterrupt',uint8(0),'isChannelwise',uint8(0)),'IOBoardType','INTLIB','UnitType','TTASSIGN','Identifier','TTASSIGN','DialogType','SL','BlockSet','NONE','SlaveProcessor','NONE','RelationId',struct('TH',struct('BlockId','TTASSIGN'))))
  wires:
  DSc/1 -> DS1104SL_DSP_PWM/3
  DSe/1 -> DS1104SL_DSP_PWM2/1
  DSa/1 -> DS1104SL_DSP_PWM/1
  DSb/1 -> DS1104SL_DSP_PWM/2
  DSd/1 -> DS1104SL_DSP_PWM/4
  DS1104SLAVE_PWMINT1/1 -> Timer Task Assignment/1

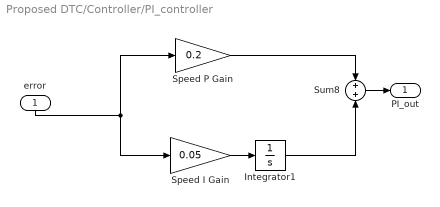
== system Proposed DTC/Controller/PI_controller ==
  error : Inport
  Integrator1 : Integrator  LimitOutput=on  UpperSaturationLimit=14  LowerSaturationLimit=-14
  Speed I Gain : Gain  Gain=0.05  SampleTime=Ts
  Speed P Gain : Gain  Gain=0.2  SampleTime=Ts
  Sum8 : Sum  SampleTime=Ts
  PI_out : Outport
  wires:
  Speed I Gain/1 -> Integrator1/1
  Integrator1/1 -> Sum8/2
  Speed P Gain/1 -> Sum8/1
  error/1 -> Speed P Gain/1, Speed I Gain/1
  Sum8/1 -> PI_out/1

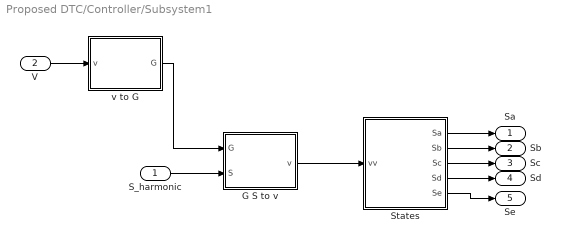
== system Proposed DTC/Controller/Subsystem1 ==
  S_harmonic : Inport
  V : Inport  Port=2
  "G S to v  " : MATLAB Function  TreatAsAtomicUnit=on
  States : MATLAB Function  TreatAsAtomicUnit=on
  v to G : MATLAB Function  TreatAsAtomicUnit=on
  Sa : Outport
  Sb : Outport  Port=2
  Sc : Outport  Port=3
  Sd : Outport  Port=4
  Se : Outport  Port=5
  wires:
  S_harmonic/1 -> "G S to v  "/2(S)
  v to G/1(G) -> "G S to v  "/1(G)
  States/1(Sa) -> Sa/1
  States/2(Sb) -> Sb/1
  States/3(Sc) -> Sc/1
  States/4(Sd) -> Sd/1
  States/5(Se) -> Se/1
  V/1 -> v to G/1(v)
  "G S to v  "/1(v) -> States/1(vv)

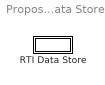
== system Proposed DTC/RTI Data/RTI Data Store ==
  RTI Data Store : Subsystem  mask(RTI_DATA_STORE){}
      mask help:
      | RTI Data Store Block. This block is used by RTI to store internal model dependent data. Deleting this block will result in data loss.
      |
      | NEVER DELETE, COPY, OR MODIFY THIS BLOCK!
      mask Help:
      | RTI Data Store Block. This block is used by RTI to store internal model dependent data. Deleting this block will result in data loss.
      | 
      | NEVER DELETE, COPY, OR MODIFY THIS BLOCK!
      mask Display: text(0.5, 0.5, ' ', 'HorizontalAlignment', 'center');

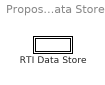
== system Proposed DTC/RTI Data/RTI Data Store/RTI Data Store ==
  RTI Data Store : Subsystem  mask(RTI_DATA_STORE){}
      mask help:
      | RTI Data Store Block. This block is used by RTI to store internal model dependent data. Deleting this block will result in data loss.
      |
      | NEVER DELETE, COPY, OR MODIFY THIS BLOCK!
      mask Help:
      | RTI Data Store Block. This block is used by RTI to store internal model dependent data. Deleting this block will result in data loss.
      | 
      | NEVER DELETE, COPY, OR MODIFY THIS BLOCK!
      mask Display: text(0.5, 0.5, ' ', 'HorizontalAlignment', 'center');

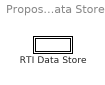
== system Proposed DTC/RTI Data/RTI Data Store/RTI Data Store/RTI Data Store ==
  RTI Data Store : Subsystem  mask(RTI_DATA_STORE){}
      mask help:
      | RTI Data Store Block. This block is used by RTI to store internal model dependent data. Deleting this block will result in data loss.
      |
      | NEVER DELETE, COPY, OR MODIFY THIS BLOCK!
      mask Help:
      | RTI Data Store Block. This block is used by RTI to store internal model dependent data. Deleting this block will result in data loss.
      | 
      | NEVER DELETE, COPY, OR MODIFY THIS BLOCK!
      mask Display: text(0.5, 0.5, ' ', 'HorizontalAlignment', 'center');

== system Proposed DTC/RTI Data/RTI Data Store/RTI Data Store/RTI Data Store/RTI Data Store ==
